simulink subsystem "ID"  (R2024b)
settings: Solver=VariableStepAuto  StartTime=0.0  StopTime=10.0  RelTol=1e-3
values from neighbouring files (symbols this model uses):
  modelStopCondition = "tohost"    [initSimuRISC.m]
libraries: hdlsllib x23, simulink x4
settings Model: Creator=stefano  LastModifiedBy=stefano

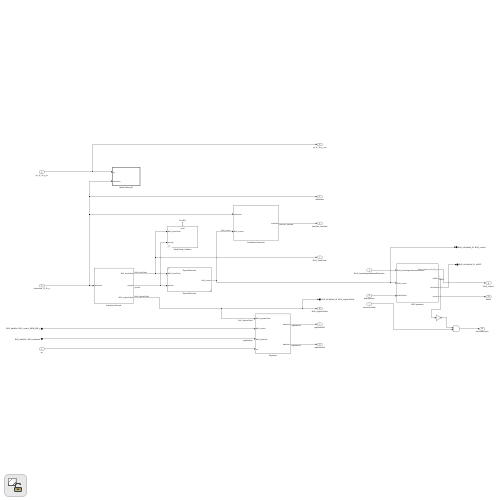
[thumbnail: Simulink's stored preview of the top-level diagram]
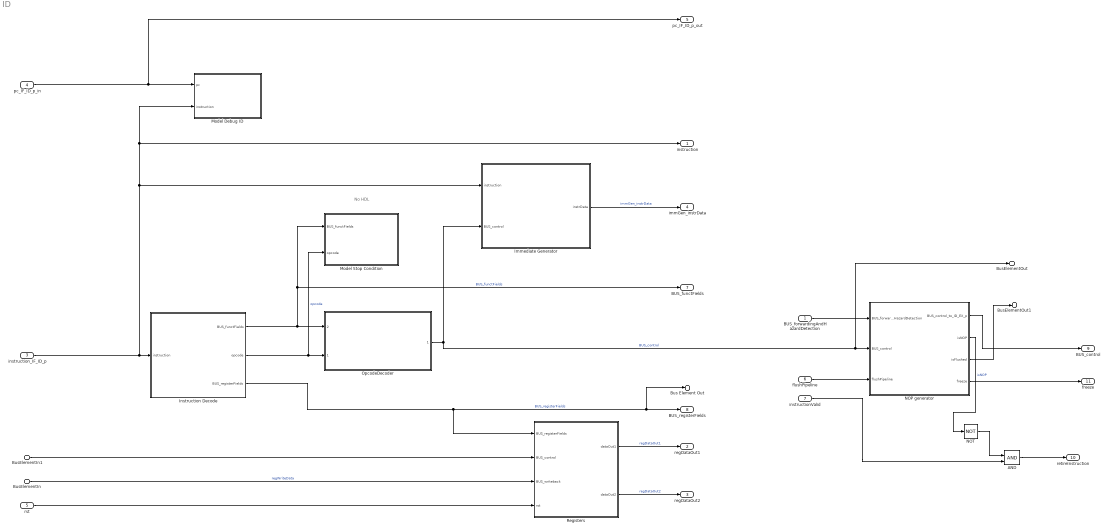
== system ID ==
  note: No HDL
  BUS_forwardingAndHazardDetection : Inport
  BusElementIn : Inport  Port=2  PortName=BUS_dataRtn  Element=BUS_writeback
  BusElementIn1 : Inport  Port=2  PortName=BUS_dataRtn  Element=BUS_control_MEM_WB_p
  instruction_IF_ID_p : Inport  Port=3
  pc_IF_ID_p_in : Inport  Port=4
  rst : Inport  Port=5
  flushPipeline : Inport  Port=6
  instructionValid : Inport  Port=7
  AND : Logic  IconShape=distinctive  AllPortsSameDT=off  OutDataTypeStr=boolean
  Immediate Generator : Subsystem
  Instruction Decode : Subsystem
  Model Debug ID : Subsystem  TreatAsAtomicUnit=on
  Model Stop Condition : Subsystem  Variant=on  VariantControl=Subsystem  AllowZeroVariantControls=on
  NOP generator : Subsystem
  NOT : Logic  Operator=NOT  IconShape=distinctive  AllPortsSameDT=off  OutDataTypeStr=boolean
  OpcodeDecoder : Subsystem  ReferencedSubsystem=OpcodeDecoder
      settings: PortSchema="{\"entries\":[{\"content\":{\"sides\":[{\"content\":{\"connectorIds\":[\"In2\",\"In1\"]},\"type\":\"ConnectorPlacement.EquallySpacedRectSide\",\"uuid\":\"b86b8d7a-0132-4aca-a0a0-24de68462b4d\"},{\"content\":{\"connectorIds\":[\"Out1\"],\"side\":\"RIGHT\"},\"type\":\"ConnectorPlacement.EquallySpacedRectSide\",\"uuid\":\"b197b565-9fcc-4bf1-9065-f309956b69ca\"},{\"content\":{\"side\":\"TOP\"},\"type\":\"ConnectorPlacement.EquallySpacedRectSide\",\"uuid\":\"9eeba0d5-f437-4f16-9295-501c529559c7\"}]},\"type\":\"ConnectorPlacement.EquallySpacedConnector\",\"uuid\":\"d2ecfa82-9cfe-4de1-8f2a-d595699d966f\"}],\"packageUris\":[\"http://schema.mathworks.com/mf0/Connector/R2020b\"],\"version\":\"1.0\"}"
  Registers : Subsystem
  instruction : Outport
  regDataOut1 : Outport  Port=2
  regDataOut2 : Outport  Port=3
  immGen_instrData : Outport  Port=4
  pc_IF_ID_p_out : Outport  Port=5
  Bus Element Out : Outport  Port=6  PortName=BUS_toFwdUnit_ID  Element=BUS_registerFields
  BusElementOut : Outport  Port=6  PortName=BUS_toFwdUnit_ID  Element=BUS_control
  BusElementOut1 : Outport  Port=6  PortName=BUS_toFwdUnit_ID  Element=isNOP
  BUS_functFields : Outport  Port=7
  BUS_registerFields : Outport  Port=8
  BUS_control : Outport  Port=9
  retireInstruction : Outport  Port=10
  freeze : Outport  Port=11
  wires:
  Registers/2(dataOut2) -> regDataOut2/1  "regDataOut2"
  Immediate Generator/1(instrData) -> immGen_instrData/1  "immGen_instrData"
  Registers/1(dataOut1) -> regDataOut1/1  "regDataOut1"
  OpcodeDecoder/1 -> NOP generator/2(BUS_control), BusElementOut/1, Immediate Generator/2(BUS_control)  "BUS_control"
  Instruction Decode/3(BUS_registerFields) -> Bus Element Out/1, BUS_registerFields/1, Registers/1(BUS_registerFields)  "BUS_registerFields"
  instruction_IF_ID_p/1 -> Instruction Decode/1(instruction), Immediate Generator/1(instruction), instruction/1, Model Debug ID/2(instruction)
  rst/1 -> Registers/4(rst)
  pc_IF_ID_p_in/1 -> Model Debug ID/1(pc), pc_IF_ID_p_out/1
  Instruction Decode/2(opcode) -> OpcodeDecoder/1, Model Stop Condition/2(opcode)  "opcode"
  BusElementIn1/1 -> Registers/2(BUS_control)
  Instruction Decode/1(BUS_functFields) -> BUS_functFields/1, Model Stop Condition/1(BUS_functFields), OpcodeDecoder/2  "BUS_functFields"
  BusElementIn/1 -> Registers/3(BUS_writeback)  "regWriteData"
  BUS_forwardingAndHazardDetection/1 -> NOP generator/1(BUS_forwardingAndHazardDetection)
  flushPipeline/1 -> NOP generator/3(flushPipeline)
  NOT/1 -> AND/1
  instructionValid/1 -> AND/2
  NOP generator/1(BUS_control_to_ID_EX_p) -> BUS_control/1
  AND/1 -> retireInstruction/1
  NOP generator/2(isNOP) -> NOT/1  "isNOP"
  NOP generator/3(isFlushed) -> BusElementOut1/1
  NOP generator/4(freeze) -> freeze/1

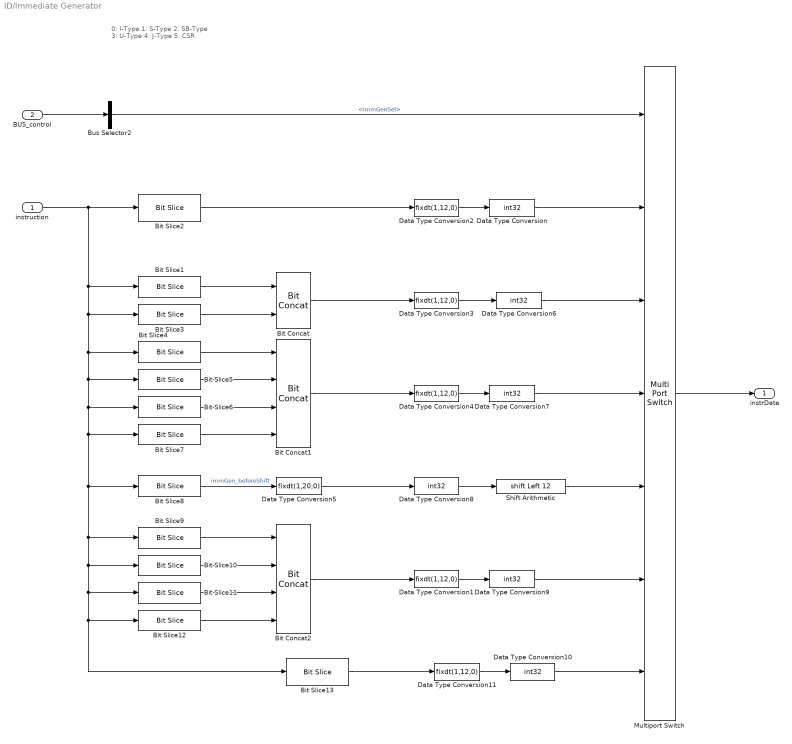
== system ID/Immediate Generator ==
  note: 0: I-Type
      | 1: S-Type
      | 2: SB-Type
      | 3: U-Type
      | 4: J-Type
      | 5: CSR
  instruction : Inport
  BUS_control : Inport  Port=2
  Bit Concat : hdlsllib/Logic and Bit Operations/Bit Concat  numInputs=2
  Bit Concat1 : hdlsllib/Logic and Bit Operations/Bit Concat  numInputs=4
  Bit Concat2 : hdlsllib/Logic and Bit Operations/Bit Concat  numInputs=4
  Bit Slice1 : hdlsllib/Logic and Bit Operations/Bit Slice  lidx=31  ridx=25
  Bit Slice10 : hdlsllib/Logic and Bit Operations/Bit Slice  lidx=19  ridx=12
  Bit Slice11 : hdlsllib/Logic and Bit Operations/Bit Slice  lidx=20  ridx=20
  Bit Slice12 : hdlsllib/Logic and Bit Operations/Bit Slice  lidx=30  ridx=21
  Bit Slice13 : hdlsllib/Logic and Bit Operations/Bit Slice  lidx=19  ridx=15
  Bit Slice2 : hdlsllib/Logic and Bit Operations/Bit Slice  lidx=31  ridx=20
  Bit Slice3 : hdlsllib/Logic and Bit Operations/Bit Slice  lidx=11  ridx=7
  Bit Slice4 : hdlsllib/Logic and Bit Operations/Bit Slice  lidx=31  ridx=31
  Bit Slice5 : hdlsllib/Logic and Bit Operations/Bit Slice  lidx=7  ridx=7
  Bit Slice6 : hdlsllib/Logic and Bit Operations/Bit Slice  lidx=30  ridx=25
  Bit Slice7 : hdlsllib/Logic and Bit Operations/Bit Slice  lidx=11  ridx=8
  Bit Slice8 : hdlsllib/Logic and Bit Operations/Bit Slice  lidx=31  ridx=12
  Bit Slice9 : hdlsllib/Logic and Bit Operations/Bit Slice  lidx=31  ridx=31
  Bus Selector2 : BusSelector  OutputSignals=immGenSel
  Data Type Conversion{,6..10} (6 alike) : DataTypeConversion  OutDataTypeStr=int32  SaturateOnIntegerOverflow=off  RndMeth=Floor
  Data Type Conversion{1..4,11} (5 alike) : DataTypeConversion  OutDataTypeStr=fixdt(1,12,0)  ConvertRealWorld=Stored Integer (SI)  SaturateOnIntegerOverflow=off  RndMeth=Floor
  Data Type Conversion5 : DataTypeConversion  OutDataTypeStr=fixdt(1,20,0)  ConvertRealWorld=Stored Integer (SI)  SaturateOnIntegerOverflow=off  RndMeth=Floor
  Multiport Switch : MultiPortSwitch  DataPortOrder=Zero-based contiguous  Inputs=6  DiagnosticForDefault=Warning  zeroidx=on  SaturateOnIntegerOverflow=off  InputSameDT=off
  Shift Arithmetic : ArithShift  BitShiftNumber=12  BitShiftDirection=Left
  instrData : Outport
  wires:
  Shift Arithmetic/1 -> Multiport Switch/5
  Data Type Conversion10/1 -> Multiport Switch/7
  Bit Slice13/1 -> Data Type Conversion11/1
  Data Type Conversion11/1 -> Data Type Conversion10/1
  Bit Concat2/1 -> Data Type Conversion1/1
  Data Type Conversion9/1 -> Multiport Switch/6
  Bit Slice10/1 -> Bit Concat2/2
  Bit Slice12/1 -> Bit Concat2/4
  Bit Slice11/1 -> Bit Concat2/3
  Data Type Conversion1/1 -> Data Type Conversion9/1
  Bit Slice9/1 -> Bit Concat2/1
  instruction/1 -> Bit Slice2/1, Bit Slice1/1, Bit Slice3/1, Bit Slice6/1, Bit Slice7/1, Bit Slice8/1, Bit Slice9/1, Bit Slice10/1, Bit Slice11/1, Bit Slice12/1, Bit Slice13/1, Bit Slice5/1, Bit Slice4/1
  Bus Selector2/1 -> Multiport Switch/1  "<immGenSel>"
  Data Type Conversion8/1 -> Shift Arithmetic/1
  Data Type Conversion7/1 -> Multiport Switch/4
  Data Type Conversion6/1 -> Multiport Switch/3
  Data Type Conversion5/1 -> Data Type Conversion8/1
  Data Type Conversion4/1 -> Data Type Conversion7/1
  Data Type Conversion3/1 -> Data Type Conversion6/1
  Data Type Conversion2/1 -> Data Type Conversion/1
  Data Type Conversion/1 -> Multiport Switch/2
  BUS_control/1 -> Bus Selector2/1
  Bit Slice8/1 -> Data Type Conversion5/1  "immGen_beforeShift"
  Bit Slice7/1 -> Bit Concat1/4
  Bit Slice6/1 -> Bit Concat1/3
  Bit Slice5/1 -> Bit Concat1/2
  Bit Slice4/1 -> Bit Concat1/1
  Multiport Switch/1 -> instrData/1
  Bit Concat1/1 -> Data Type Conversion4/1
  Bit Concat/1 -> Data Type Conversion3/1
  Bit Slice3/1 -> Bit Concat/2
  Bit Slice1/1 -> Bit Concat/1
  Bit Slice2/1 -> Data Type Conversion2/1

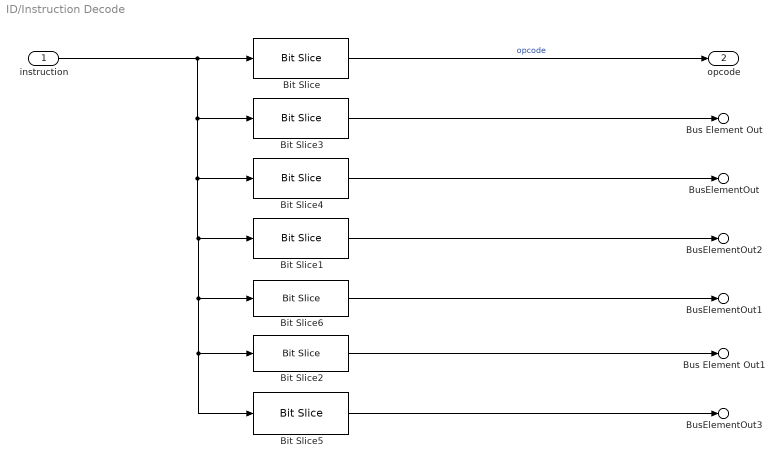
== system ID/Instruction Decode ==
  instruction : Inport
  Bit Slice : hdlsllib/Logic and Bit Operations/Bit Slice  lidx=6  ridx=0
  Bit Slice1 : hdlsllib/Logic and Bit Operations/Bit Slice  lidx=11  ridx=7
  Bit Slice2 : hdlsllib/Logic and Bit Operations/Bit Slice  lidx=14  ridx=12
  Bit Slice3 : hdlsllib/Logic and Bit Operations/Bit Slice  lidx=19  ridx=15
  Bit Slice4 : hdlsllib/Logic and Bit Operations/Bit Slice  lidx=24  ridx=20
  Bit Slice5 : hdlsllib/Logic and Bit Operations/Bit Slice  lidx=31  ridx=25
  Bit Slice6 : hdlsllib/Logic and Bit Operations/Bit Slice  lidx=31  ridx=20
  Bus Element Out1 : Outport  PortName=BUS_functFields  Element=funct3
  BusElementOut3 : Outport  PortName=BUS_functFields  Element=funct7
  opcode : Outport  Port=2
  Bus Element Out : Outport  Port=3  PortName=BUS_registerFields  Element=rs1
  BusElementOut : Outport  Port=3  PortName=BUS_registerFields  Element=rs2
  BusElementOut1 : Outport  Port=3  PortName=BUS_registerFields  Element=CSRAddr
  BusElementOut2 : Outport  Port=3  PortName=BUS_registerFields  Element=rd
  wires:
  Bit Slice6/1 -> BusElementOut1/1
  instruction/1 -> Bit Slice/1, Bit Slice3/1, Bit Slice4/1, Bit Slice1/1, Bit Slice2/1, Bit Slice5/1, Bit Slice6/1
  Bit Slice5/1 -> BusElementOut3/1
  Bit Slice4/1 -> BusElementOut/1
  Bit Slice3/1 -> Bus Element Out/1
  Bit Slice2/1 -> Bus Element Out1/1
  Bit Slice1/1 -> BusElementOut2/1
  Bit Slice/1 -> opcode/1  "opcode"

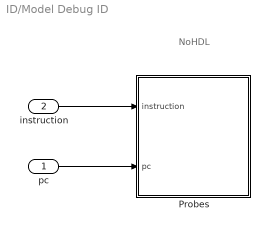
== system ID/Model Debug ID ==
  note: NoHDL
  pc : Inport
  instruction : Inport  Port=2
  Probes : Subsystem
  wires:
  pc/1 -> Probes/2(pc)
  instruction/1 -> Probes/1(instruction)

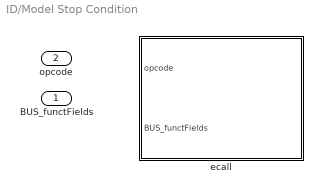
== system ID/Model Stop Condition ==
  BUS_functFields : Inport
  opcode : Inport  Port=2
  ecall : Subsystem  VariantControl="strcmp(modelStopCondition, \"ecall\")"

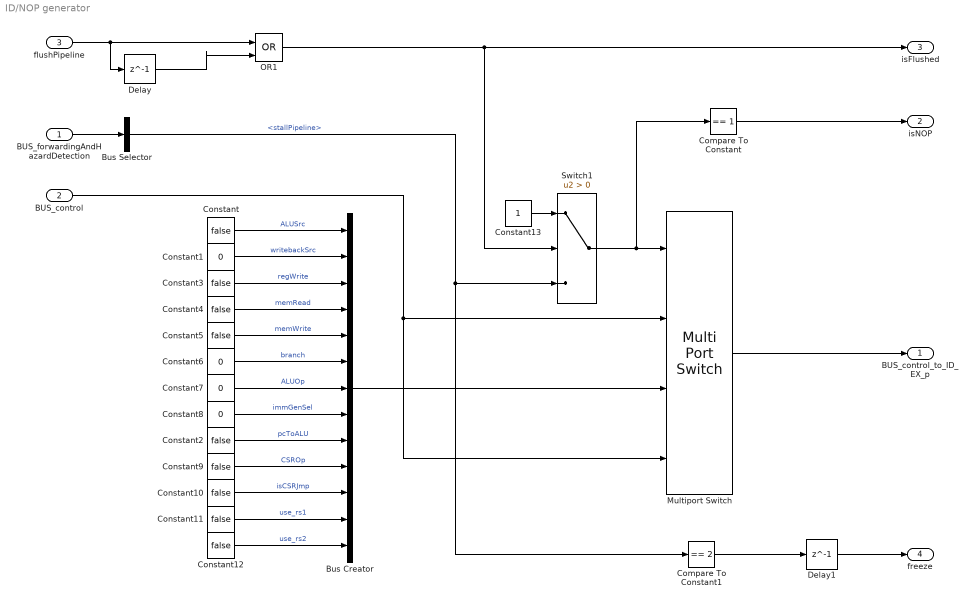
== system ID/NOP generator ==
  BUS_forwardingAndHazardDetection : Inport
  BUS_control : Inport  Port=2
  flushPipeline : Inport  Port=3
  Bus Creator : BusCreator  Inputs=13
  Bus Selector : BusSelector  OutputSignals=stallPipeline
  Compare To Constant : simulink/Logic and Bit Operations/Compare To Constant  relop===  const=1  OutDataTypeStr=boolean
  Compare To Constant1 : simulink/Logic and Bit Operations/Compare To Constant  relop===  const=2  OutDataTypeStr=boolean
  Constant{,2..5,9..12} (9 alike) : Constant  Value=false  SampleTime=-1
  Constant1 : Constant  Value=0  OutDataTypeStr=fixdt(0,2,0)  SampleTime=-1
  Constant13 : Constant  OutDataTypeStr=fixdt(0,2,0)  SampleTime=-1
  Constant6 : Constant  Value=0  OutDataTypeStr=fixdt(0,3,0)  SampleTime=-1
  Constant7 : Constant  Value=0  OutDataTypeStr=fixdt(0,3,0)  SampleTime=-1
  Constant8 : Constant  Value=0  OutDataTypeStr=uint8  SampleTime=-1
  Delay : Delay  DelayLength=1
  Delay1 : Delay  DelayLength=1
  Multiport Switch : MultiPortSwitch  DataPortOrder=Zero-based contiguous  zeroidx=on  SaturateOnIntegerOverflow=off  InputSameDT=off
  OR1 : Logic  Operator=OR  IconShape=distinctive  AllPortsSameDT=off  OutDataTypeStr=boolean
  Switch1 : Switch  Criteria=u2 > Threshold  SaturateOnIntegerOverflow=off  InputSameDT=off
  BUS_control_to_ID_EX_p : Outport
  isNOP : Outport  Port=2
  isFlushed : Outport  Port=3
  freeze : Outport  Port=4
  wires:
  Delay1/1 -> freeze/1
  Compare To Constant1/1 -> Delay1/1
  BUS_control/1 -> Multiport Switch/2, Multiport Switch/4
  Bus Creator/1 -> Multiport Switch/3
  Compare To Constant/1 -> isNOP/1
  Switch1/1 -> Multiport Switch/1, Compare To Constant/1
  Constant13/1 -> Switch1/1
  BUS_forwardingAndHazardDetection/1 -> Bus Selector/1
  Bus Selector/1 -> Switch1/3, Compare To Constant1/1  "<stallPipeline>"
  Delay/1 -> OR1/2
  flushPipeline/1 -> OR1/1, Delay/1
  OR1/1 -> isFlushed/1, Switch1/2
  Constant12/1 -> Bus Creator/13  "use_rs2"
  Constant11/1 -> Bus Creator/12  "use_rs1"
  Constant8/1 -> Bus Creator/8  "immGenSel"
  Constant5/1 -> Bus Creator/5  "memWrite"
  Constant4/1 -> Bus Creator/4  "memRead"
  Constant3/1 -> Bus Creator/3  "regWrite"
  Constant1/1 -> Bus Creator/2  "writebackSrc"
  Constant10/1 -> Bus Creator/11  "isCSRJmp"
  Constant9/1 -> Bus Creator/10  "CSROp"
  Constant2/1 -> Bus Creator/9  "pcToALU"
  Constant7/1 -> Bus Creator/7  "ALUOp"
  Constant6/1 -> Bus Creator/6  "branch"
  Constant/1 -> Bus Creator/1  "ALUSrc"
  Multiport Switch/1 -> BUS_control_to_ID_EX_p/1

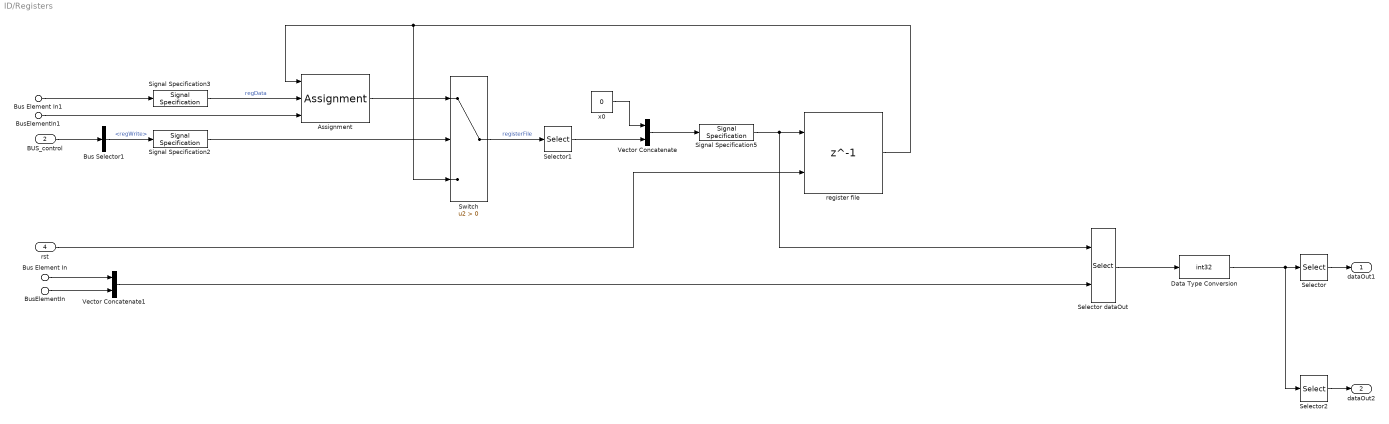
== system ID/Registers ==
  Bus Element In : Inport  PortName=BUS_registerFields  Element=rs1
  BusElementIn : Inport  PortName=BUS_registerFields  Element=rs2
  BUS_control : Inport  Port=2
  BusElementIn1 : Inport  Port=3  PortName=BUS_writeback  Element=rd
  Bus Element In1 : Inport  Port=3  PortName=BUS_writeback  Element=regWriteData
  rst : Inport  Port=4
  Assignment : Assignment  IndexMode=Zero-based  DiagnosticForDimensions=Warning  IndexOptions=Index vector (port)  Indices=1  OutputSizes=1
  Bus Selector1 : BusSelector  OutputSignals=regWrite
  Data Type Conversion : DataTypeConversion  OutDataTypeStr=int32  ConvertRealWorld=Stored Integer (SI)  SaturateOnIntegerOverflow=off  RndMeth=Floor
  Selector : Selector  InputPortWidth=2  IndexOptions=Index vector (dialog)  Indices=1  OutputSizes=1
  Selector dataOut : Selector  IndexMode=Zero-based  InputPortWidth=32  IndexOptions=Index vector (port)  Indices=[1 3]  OutputSizes=1
  Selector1 : Selector  InputPortWidth=32  IndexOptions=Index vector (dialog)  Indices=2:32  OutputSizes=1
  Selector2 : Selector  InputPortWidth=2  IndexOptions=Index vector (dialog)  Indices=2  OutputSizes=1
  Signal Specification2 : SignalSpecification  OutDataTypeStr=boolean
  Signal Specification3 : SignalSpecification  OutDataTypeStr=uint32
  Signal Specification5 : SignalSpecification  OutDataTypeStr=uint32  Dimensions=32
  Switch : Switch  Criteria=u2 > Threshold  SaturateOnIntegerOverflow=off  InputSameDT=off
  Vector Concatenate : Concatenate
  Vector Concatenate1 : Concatenate
  register file : Delay  DelayLength=1  InitialCondition=uint32(zeros(32,1))  ExternalReset=Level hold
      settings: InputPortMap=u0,r5
  x0 : Constant  Value=0  OutDataTypeStr=registerDataType  SampleTime=-1
  dataOut1 : Outport
  dataOut2 : Outport  Port=2
  wires:
  Selector2/1 -> dataOut2/1
  Selector/1 -> dataOut1/1
  Vector Concatenate1/1 -> Selector dataOut/2
  Vector Concatenate/1 -> Signal Specification5/1
  BusElementIn1/1 -> Assignment/3
  Bus Element In1/1 -> Signal Specification3/1
  Signal Specification5/1 -> register file/1, Selector dataOut/1
  Signal Specification3/1 -> Assignment/2  "regData"
  Selector1/1 -> Vector Concatenate/2
  Assignment/1 -> Switch/1
  Bus Selector1/1 -> Signal Specification2/1  "<regWrite>"
  Data Type Conversion/1 -> Selector/1, Selector2/1
  Bus Element In/1 -> Vector Concatenate1/1
  Signal Specification2/1 -> Switch/2
  Switch/1 -> Selector1/1  "registerFile"
  BUS_control/1 -> Bus Selector1/1
  BusElementIn/1 -> Vector Concatenate1/2
  x0/1 -> Vector Concatenate/1
  rst/1 -> register file/2
  Selector dataOut/1 -> Data Type Conversion/1
  register file/1 -> Assignment/1, Switch/3

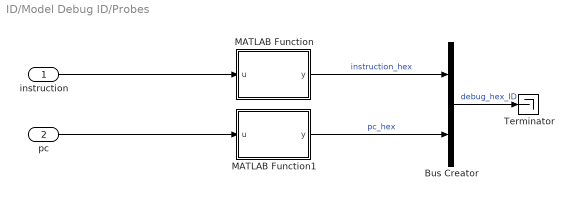
== system ID/Model Debug ID/Probes ==
  instruction : Inport
  pc : Inport  Port=2
  Bus Creator : BusCreator  Inputs=2
  MATLAB Function : MATLAB Function  TreatAsAtomicUnit=on
  MATLAB Function1 : MATLAB Function  TreatAsAtomicUnit=on
  Terminator : Terminator
  wires:
  MATLAB Function1/1(y) -> Bus Creator/2  "pc_hex"
  Bus Creator/1 -> Terminator/1  "debug_hex_ID"
  instruction/1 -> MATLAB Function/1(u)
  pc/1 -> MATLAB Function1/1(u)
  MATLAB Function/1(y) -> Bus Creator/1  "instruction_hex"

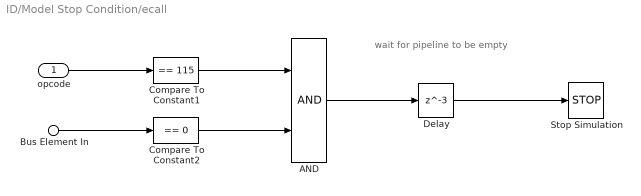
== system ID/Model Stop Condition/ecall ==
  note: wait for pipeline to be empty
  opcode : Inport
  Bus Element In : Inport  Port=2  PortName=BUS_functFields  Element=funct3
  AND : Logic  IconShape=distinctive  AllPortsSameDT=off  OutDataTypeStr=boolean
  Compare To Constant1 : simulink/Logic and Bit Operations/Compare To Constant  relop===  const=115  OutDataTypeStr=boolean
  Compare To Constant2 : simulink/Logic and Bit Operations/Compare To Constant  relop===  const=0  OutDataTypeStr=boolean
  Delay : Delay  DelayLength=3
  Stop Simulation : Stop
  wires:
  Compare To Constant2/1 -> AND/2
  Delay/1 -> Stop Simulation/1
  Bus Element In/1 -> Compare To Constant2/1
  opcode/1 -> Compare To Constant1/1
  AND/1 -> Delay/1
  Compare To Constant1/1 -> AND/1

== matlab function ID/Model Debug ID/Probes/MATLAB Function1 ==
  data: u input; y output string
function y = toHex(u)

y = string(dec2hex(u, 8));

== matlab function ID/Model Debug ID/Probes/MATLAB Function ==
  data: u input; y output string
function y = toHex(u)

y = string(dec2hex(u, 8));
